simulink model "Motor_Model_DDPG"  (R2022a)
settings: Solver=FixedStepAuto  StartTime=0.0  StopTime=inf  FixedStep=Ts  RelTol=1e-3
values from neighbouring files (symbols this model uses):
  b = 0.1    [ddpg.m]
  J = 0.1    [ddpg.m]
  K = 0.11    [ddpg.m]
  L = 0.5    [ddpg.m]
  R = 1    [ddpg.m]
  Ts = 0.1    [ddpg.m]
libraries: rllib x1
settings Model: Creator=sansh  LastModifiedBy=cran
settings SolverCC: AlgebraicLoopSolver=TrustRegion
settings DebuggingCC: UnconnectedInputMsg=warning  UnconnectedOutputMsg=warning  UnconnectedLineMsg=warning  SFMachineParentedDataDiag=warning  ArithmeticOperatorsInVariantConditions=warning
settings SFSimCC: SimUseLocalCustomCode=off  CustomCodeUndefinedFunction=UseInterfaceOnly
settings RTWCC: RTWUseLocalCustomCode=off
settings CodeAppCC: StateflowObjectComments=on

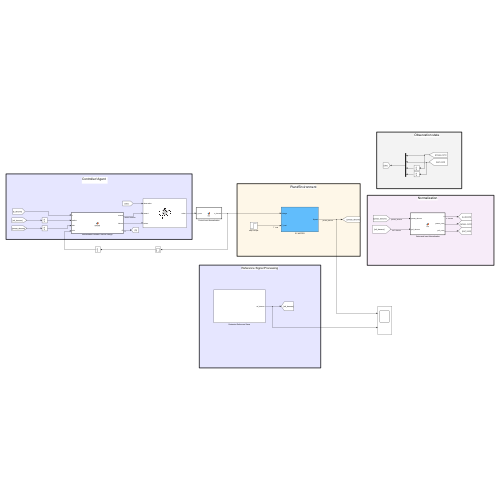
[thumbnail: Simulink's stored preview of the top-level diagram]
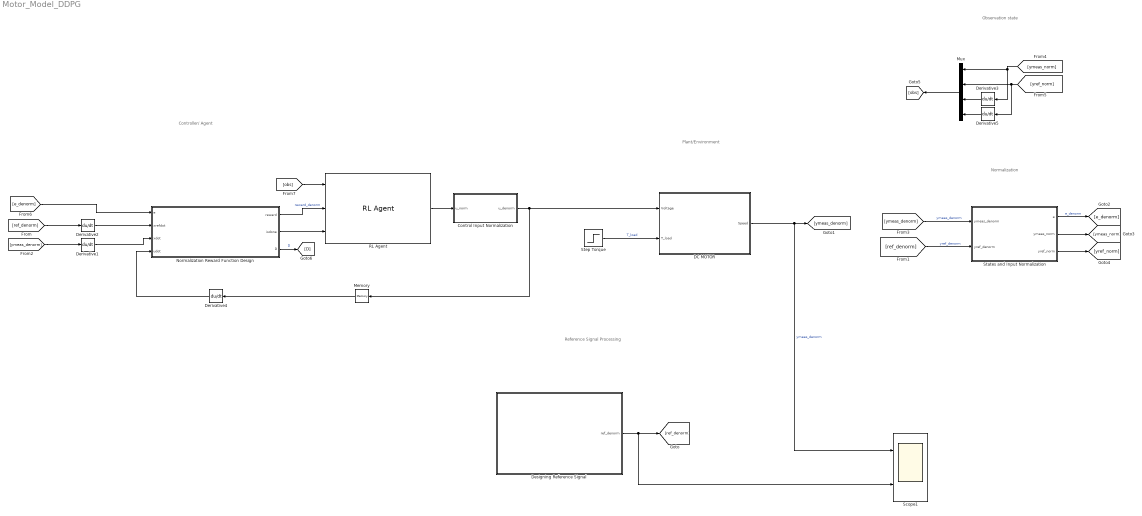
== system Motor_Model_DDPG ==
  note: Reference Signal Processing
  note: Normalization
  note: Plant/Environment
  note: Observation state
  note: Controller/ Agent
  Control Input Normalization : MATLAB Function  TreatAsAtomicUnit=on
  DC MOTOR : Subsystem
  Derivative{1..5} (5 alike) : Derivative
  Designing Reference Signal : Subsystem
  Memory : Memory
  Mux : Mux
  Normalization Reward Function Design : MATLAB Function  TreatAsAtomicUnit=on
  RL Agent : rllib/RL Agent  Agent=agent  ExternalActionAsInput=off  ProvideLastAction=off  ProvideCumRwd=off  TreatAsDirectFeedthrough=on  UseStrictObservationDataTypes=off
  Scope1 : Scope  NumInputPorts=2
  States and Input Normalization : MATLAB Function  TreatAsAtomicUnit=on
  Step Torque : Step  Time=0  After=0  SampleTime=Ts
  wires:
  Normalization Reward Function Design/2(isdone) -> RL Agent/3
  DC MOTOR/1(Speed) -> Scope1/1, [ymeas_denorm]  "ymeas_denorm"
  Step Torque/1 -> DC MOTOR/2(T_load)  "T_load"
  RL Agent/1 -> Control Input Normalization/1(u_norm)
  Memory/1 -> Derivative4/1
  Derivative4/1 -> Normalization Reward Function Design/4(udot)
  Control Input Normalization/1(u_denorm) -> Memory/1, DC MOTOR/1(Voltage)
  Designing Reference Signal/1(ref_denorm) -> Scope1/2, [ref_denorm]
  [ref_denorm] -> Derivative2/1
  Derivative2/1 -> Normalization Reward Function Design/2(xrefdot)
  [ref_denorm] -> States and Input Normalization/2(yref_denorm)  "yref_denorm"
  [ymeas_denorm] -> Derivative1/1
  Derivative1/1 -> Normalization Reward Function Design/3(xdot)
  States and Input Normalization/1(e) -> [e_denorm]  "e_denorm"
  States and Input Normalization/2(ymeas_norm) -> [ymeas_norm]
  States and Input Normalization/3(yref_norm) -> [yref_norm]
  [ymeas_denorm] -> States and Input Normalization/1(ymeas_denorm)  "ymeas_denorm"
  Normalization Reward Function Design/1(reward) -> RL Agent/2  "reward_denorm"
  [ymeas_norm] -> Derivative3/1, Mux/1
  [yref_norm] -> Derivative5/1, Mux/2
  Mux/1 -> [obs]
  [e_denorm] -> Normalization Reward Function Design/1(e)
  [obs] -> RL Agent/1
  Normalization Reward Function Design/3(D) -> [D]  "D"
  Derivative3/1 -> Mux/3
  Derivative5/1 -> Mux/4

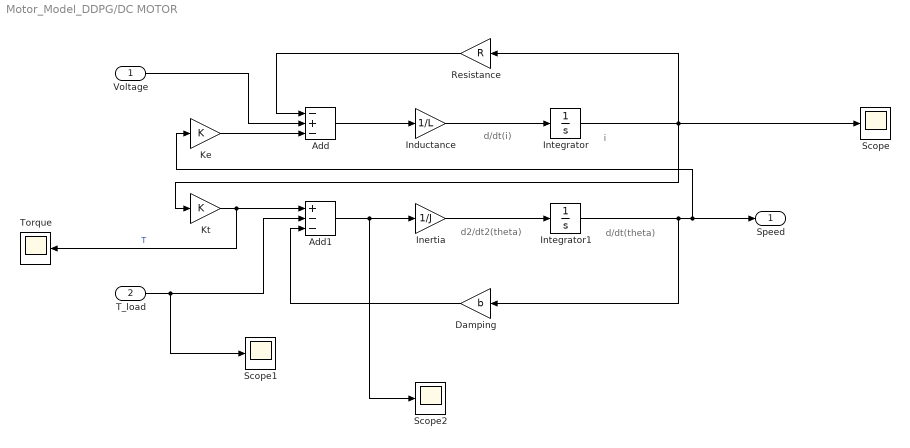
== system Motor_Model_DDPG/DC MOTOR ==
  note: i
  note: d/dt(i)
  note: d/dt(theta)
  note: d2/dt2(theta)
  Voltage : Inport
  T_load : Inport  Port=2
  Add : Sum  Inputs=-+-
  Add1 : Sum  Inputs=+--
  Damping : Gain  Gain=b
  Inductance : Gain  Gain=1/L
  Inertia : Gain  Gain=1/J
  Integrator : Integrator
  Integrator1 : Integrator
  Ke : Gain  Gain=K
  Kt : Gain  Gain=K
  Resistance : Gain  Gain=R
  Scope : Scope
  Scope1 : Scope
  Scope2 : Scope
  Torque : Scope
  Speed : Outport
  wires:
  Inductance/1 -> Integrator/1
  Integrator1/1 -> Damping/1, Speed/1, Ke/1
  Inertia/1 -> Integrator1/1
  Integrator/1 -> Scope/1, Resistance/1, Kt/1
  Kt/1 -> Torque/1, Add1/1  "T"
  Voltage/1 -> Add/2
  Resistance/1 -> Add/1
  Damping/1 -> Add1/3
  Ke/1 -> Add/3
  Add/1 -> Inductance/1
  Add1/1 -> Scope2/1, Inertia/1
  T_load/1 -> Scope1/1, Add1/2

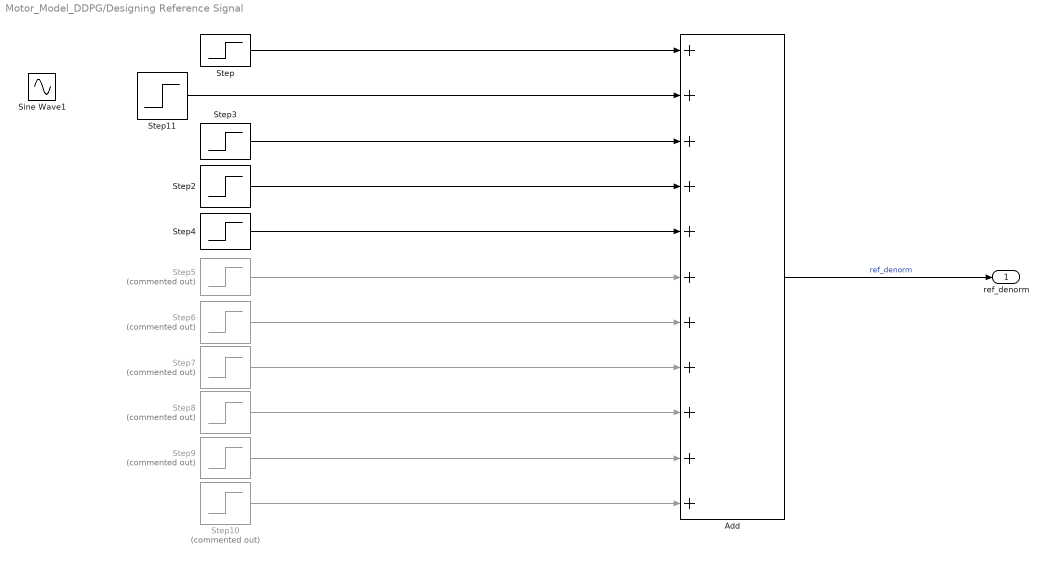
== system Motor_Model_DDPG/Designing Reference Signal ==
  Add : Sum  Inputs=+++++++++++
  Sine Wave1 : Sin  SampleTime=0
  Step : Step  Time=0  SampleTime=Ts
  Step10 : Step  Commented=on  Time=0  After=0  SampleTime=0
  Step11 : Step  Time=12  SampleTime=Ts
  Step2 : Step  Time=36  SampleTime=Ts
  Step3 : Step  Time=24  After=2  SampleTime=Ts
  Step4 : Step  Time=48  SampleTime=Ts
  Step5 : Step  Commented=on  Time=50  SampleTime=Ts
  Step6 : Step  Commented=on  Time=10  After=7  SampleTime=Ts
  Step7 : Step  Commented=on  Time=86  SampleTime=Ts
  Step8 : Step  Commented=on  Time=160  After=0  SampleTime=Ts
  Step9 : Step  Commented=on  Time=180  After=0  SampleTime=Ts
  ref_denorm : Outport
  wires:
  Step/1 -> Add/1
  Step5/1 -> Add/6
  Step2/1 -> Add/4
  Step10/1 -> Add/11
  Step8/1 -> Add/9
  Step6/1 -> Add/7
  Step9/1 -> Add/10
  Step7/1 -> Add/8
  Step11/1 -> Add/2
  Step3/1 -> Add/3
  Step4/1 -> Add/5
  Add/1 -> ref_denorm/1  "ref_denorm"

== matlab function Motor_Model_DDPG/Normalization Reward Function Design ==
  data: e input; xrefdot input; reward output; isdone output; xdot input; D output; udot input
function [reward,isdone,D] = reward(e,xrefdot,xdot,udot)


if (e<=0.02)&&(e>-0.02)
    D = 100;
else 
    D = 0;
end

e_dot = xrefdot-xdot;

% Designing Reward Function 
reward =-6*abs(e)-0.01*abs(xdot)+D;

% done if succeeded the convergence
% isdone = madeit
isdone = 0;

== matlab function Motor_Model_DDPG/Control Input Normalization ==
  data: u_norm input; u_denorm output
function u_denorm = fcn(u_norm)

u_max = 10;
u_min = 0;

% Normalize formula

% x_norm = 2*[(x - min)/(max - min)] - 1;

% Denormalize formula 

u_denorm = [u_norm*(u_max-u_min)+u_max+u_min]/2;

== matlab function Motor_Model_DDPG/States and Input Normalization ==
  data: ymeas_denorm input; e output; yref_denorm input; ymeas_norm output; yref_norm output
%fuction to narmalize the mesurement generated by the system and the
%reference trajectory
function [e,ymeas_norm,yref_norm] = fcn(ymeas_denorm,yref_denorm)

ymeas_max = 8; % (ymeas_48V  + white noise)
ymeas_min = 0; % (ymeas_0V - white noise)

yref_max = 6;
yref_min = 0;

%  Normalizing between [-1,1]

ymeas_norm = (2*(ymeas_denorm - ymeas_min)/(ymeas_max - ymeas_min)-1);
yref_norm = (2*(yref_denorm - yref_min)/(yref_max - yref_min)-1);
% 
% e = yref_denorm - ymeas_denorm;
% 
% 

e = yref_denorm - ymeas_denorm;
% 
% 
% if (e<=0.05)&&(e>-0.05)
%     D = 0;
% else 
%     D = 1;
% end


end
